simulink model "q2_trim_modelo24a"  (R2024a)
settings: Solver=VariableStepAuto  StartTime=0.0  StopTime=10  RelTol=1e-3
values from neighbouring files (symbols this model uses):
  TrimInput = (lb+ub)/2    [trimagem_piper.m]
settings Model: Creator=anade  LastModifiedBy=pedroreid

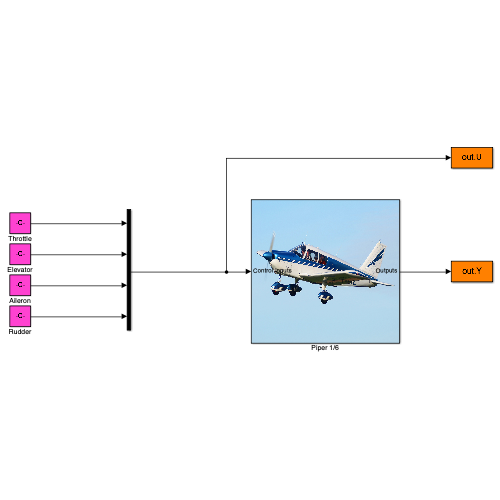
[thumbnail: Simulink's stored preview of the top-level diagram]
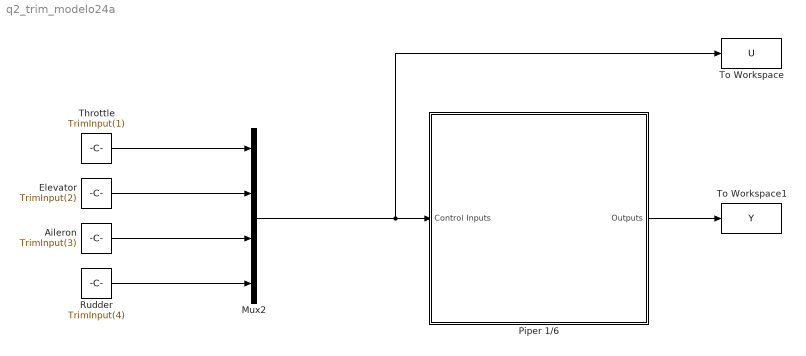
== system q2_trim_modelo24a ==
  Aileron : Constant  Value=TrimInput(3)
  Elevator : Constant  Value=TrimInput(2)
  Mux2 : Mux
  Piper 1/6 : Subsystem
      mask Display: image('piper.jpg');
  Rudder : Constant  Value=TrimInput(4)
  Throttle : Constant  Value=TrimInput(1)
  To Workspace : ToWorkspace  VariableName=U  SaveFormat=Structure With Time  SampleTime=-1
  To Workspace1 : ToWorkspace  VariableName=Y  SaveFormat=Structure With Time  SampleTime=-1
  wires:
  Throttle/1 -> Mux2/1
  Piper 1/6/1(Outputs) -> To Workspace1/1
  Mux2/1 -> To Workspace/1, Piper 1/6/1(Control Inputs)
  Elevator/1 -> Mux2/2
  Aileron/1 -> Mux2/3
  Rudder/1 -> Mux2/4

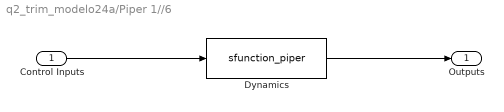
== system q2_trim_modelo24a/Piper 1//6 ==
  Control Inputs : Inport
  Dynamics : S-Function  FunctionName=sfunction_piper  Parameters=par_gen,par_aero,par_prop, Xe  SFunctionDeploymentMode=off  EnableBusSupport=off
  Outputs : Outport
  wires:
  Control Inputs/1 -> Dynamics/1
  Dynamics/1 -> Outputs/1
